simulink model "precom_dyn_1"  (Simulink 8.7)
settings: Solver=ode45  StartTime=0.0  StopTime=5  FixedStep=.001  RelTol=1e-3
values from neighbouring files (symbols this model uses):
  F1 = -acker(A,B,P1)    [Data.m]    (also in Q5.m)
  G = k*(s+c)/(s+a)/(s+b)/(s+b)    [Data.m]    (also in Q5.m)
  Gm = 1/(Tr*s+1)^3    [Data.m]
  K1 = acker(A',C',Po1)'    [Data.m]    (also in Q5.m)
  K1_ = minreal(K1_,0.0001)    [Data.m]
  S1 = 1/(1+L1)    [Data.m]    (also in Q5.m)
undefined symbols (not defined in the file or in its folder): A, B, C
libraries: cstblocks x3
settings Model: Creator=user  LastModifiedBy=NAD
settings SolverCC: ZeroCrossControl=EnableAll  PositivePriorityOrder=on
settings DataIOCC: LimitDataPoints=off  SignalLoggingSaveFormat=ModelDataLogs
settings OptimizationCC: BooleanDataType=off  InitFltsAndDblsToZero=on
settings DebuggingCC: SaveWithParameterizedLinksMsg=none  SignalResolutionControl=TryResolveAllWithWarning  MultiTaskDSMMsg=warning  MultiTaskCondExecSysMsg=none  FcnCallInpInsideContextMsg=UseLocalSettings
settings HardwareCC: TargetUnknown=on
settings GRTTargetCC: TargetFcnLib=ansi_tfl_tmw.mat  CombineOutputUpdateFcns=off  GRTInterface=on

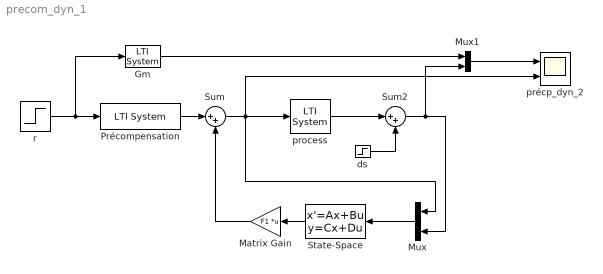
== system precom_dyn_1 ==
  Gm : cstblocks/LTI System  sys=Gm  IC=[]
  Matrix Gain : Gain  Gain=F1  Multiplication=Matrix(K*u)  SaturateOnIntegerOverflow=on  OutDataTypeStr=Inherit: Same as input  ParamDataTypeStr=Inherit: Same as input
  Mux : Mux  Inputs=2
  Mux1 : Mux  Inputs=2
  Précompensation : cstblocks/LTI System  sys=Gm/K1_/(G*S1)  IC=[]
  State-Space : StateSpace  A=A-K1*C  B=[B K1]  C=eye(3)  D=zeros(3,2)  X0=0
  Sum : Sum  Inputs=|++  SaturateOnIntegerOverflow=on  InputSameDT=on  OutDataTypeStr=Inherit: Same as first input
  Sum2 : Sum  Inputs=|++  SaturateOnIntegerOverflow=on  InputSameDT=on  OutDataTypeStr=Inherit: Same as first input
  ds : Step  Time=3  SampleTime=0
  process : cstblocks/LTI System  sys=G  IC=[]
  précp_dyn_2 : Scope  NumInputPorts=2
  r : Step  SampleTime=0
  wires:
  Mux/1 -> State-Space/1
  State-Space/1 -> Matrix Gain/1
  Matrix Gain/1 -> Sum/2
  Sum/1 -> précp_dyn_2/2, process/1, Mux/1
  Précompensation/1 -> Sum/1
  r/1 -> Précompensation/1, Gm/1
  Mux1/1 -> précp_dyn_2/1
  process/1 -> Sum2/1
  Sum2/1 -> Mux/2, Mux1/2
  ds/1 -> Sum2/2
  Gm/1 -> Mux1/1
